simulink model "PL1_P2_PositionControl"  (R2022b)
settings: Solver=VariableStepAuto  StartTime=0.0  StopTime=10.0  RelTol=1e-3
values from neighbouring files (symbols this model uses):
  refx = rand    [RunPositionControl.m]
  refy = rand    [RunPositionControl.m]
undefined symbols (not defined in the file or in its folder): DiscIntNeverNeededParam
settings Model: Creator=lucas  LastModifiedBy=lucas
settings DataIOCC: ReturnWorkspaceOutputs=off

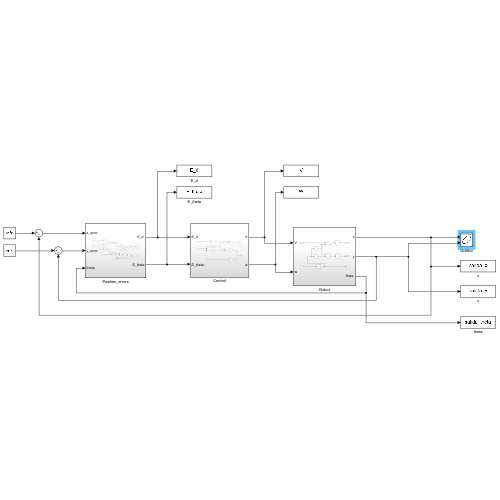
[thumbnail: Simulink's stored preview of the top-level diagram]
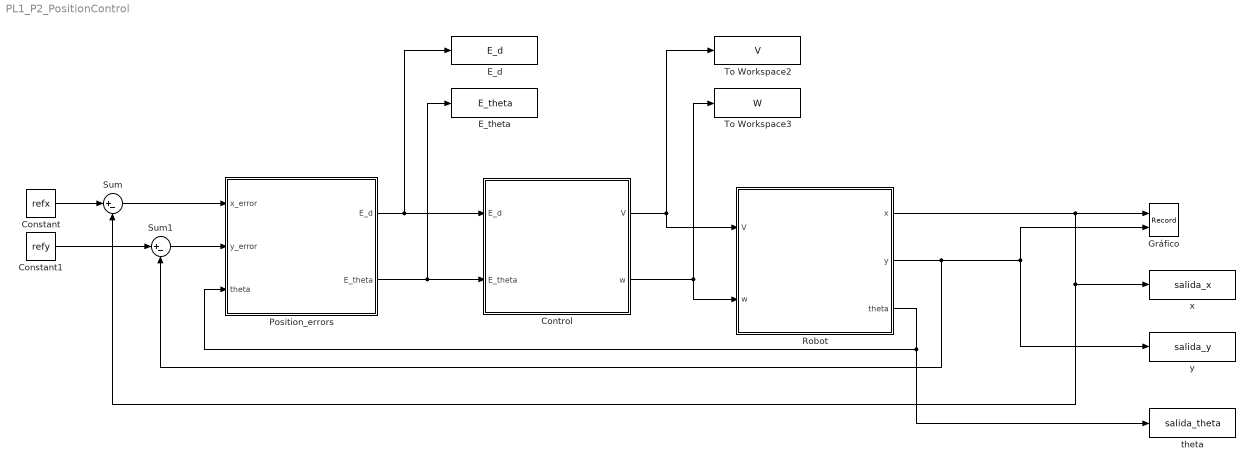
== system PL1_P2_PositionControl ==
  Constant : Constant  Value=refx
  Constant1 : Constant  Value=refy
  Control : Subsystem
  E_d : ToWorkspace  VariableName=E_d  SaveFormat=Structure With Time  SampleTime=-1
  E_theta : ToWorkspace  VariableName=E_theta  SaveFormat=Structure With Time  SampleTime=-1
  Gráfico : Record  FileSettingsInternal="{\"entries\":[{\"content\":{\"excelSettings\":{\"content\":{},\"type\":\"Streamout.ExcelSettings\"}},\"type\":\"Streamout.FileSettingStorage\",\"uuid\":\"\"}],\"packageUris\":[\"http:\\/\\/schema.mathworks.com\\/mf0\\/streamout_blocks\\/R2020a\"],\"version\":\"1.0\"}"  Layout=[1 1]  SignalsInternal="{\"entries\":[{\"content\":{\"signals\":[{\"content\":{\"blockPath\":[],\"channel\":[],\"dimensions\":[1],\"domain\":\"\",\"lineColor\":\"#0072bd\",\"plots\":[1],\"port\":1,\"sid\":[\"\"],\"signalID\":2497,\"signalName\":\"Robot:1\"},\"type\":\"RecordBlkView.Signal\",\"uuid\":\"\"},{\"content\":{\"blockPath\":[],\"channel\":[],\"dimensions\":[1],\"domain\":\"\",\"lineColor\":\"#d95319\",\"plots\":[1],\"port\":2,\"sid\":[\"\"],\"signalID\":2501,\"signalName\":\"Robot:2\"},\"type\":\"RecordBlkView.Signal\",\"uuid\":\"\"}]},\"type\":\"RecordBlkView.InputSignals\",\"uuid\":\"\"}],\"packageUris\":[\"http:\\/\\/schema.mathworks.com\\/mf0\\/streamout_blocks\\/R2020a\"],\"version\":\"1.0\"}"  VisualizationBindings="{\"xyplotplugin\":{\"info\":[{\"series\":[{\"bindingParametersList\":[{\"parameter\":\"X-Axis\",\"signalID\":2497,\"signalName\":\"Robot:1\"},{\"parameter\":\"Y-Axis\",\"signalID\":2501,\"signalName\":\"Robot:2\"}],\"seriesID\":28655},{\"bindingParametersList\":[{\"parameter\":\"X-Axis\",\"signalID\":2501,\"signalName\":\"Robot:2\"},{\"parameter\":\"Y-Axis\",\"signalID\":2497,\"signalName\":\"Robot:1\"}],\"seriesID\":47687}],\"subplotID\":1}]}}"  CompatibilityTag=XY  st=-1
  Position_errors : Subsystem
  Robot : Subsystem
  Sum : Sum  Inputs=|+-
  Sum1 : Sum  Inputs=|+-
  To Workspace2 : ToWorkspace  VariableName=V  SaveFormat=Structure With Time  SampleTime=-1
  To Workspace3 : ToWorkspace  VariableName=W  SaveFormat=Structure With Time  SampleTime=-1
  theta : ToWorkspace  VariableName=salida_theta  SaveFormat=Structure With Time  SampleTime=-1
  x : ToWorkspace  VariableName=salida_x  SaveFormat=Structure With Time  SampleTime=-1
  y : ToWorkspace  VariableName=salida_y  SaveFormat=Structure With Time  SampleTime=-1
  wires:
  Position_errors/2(E_theta) -> Control/2(E_theta), E_theta/1
  Control/2(w) -> To Workspace3/1, Robot/2(w)
  Constant1/1 -> Sum1/1
  Constant/1 -> Sum/1
  Sum/1 -> Position_errors/1("x_error ")
  Sum1/1 -> Position_errors/2("y_error ")
  Position_errors/1("E_d ") -> E_d/1, Control/1(E_d)
  Control/1(V) -> Robot/1(V), To Workspace2/1
  Robot/1(x) -> Sum/2, x/1, Gráfico/1
  Robot/2(y) -> Sum1/2, Gráfico/2, y/1
  Robot/3("theta ") -> Position_errors/3(theta), theta/1

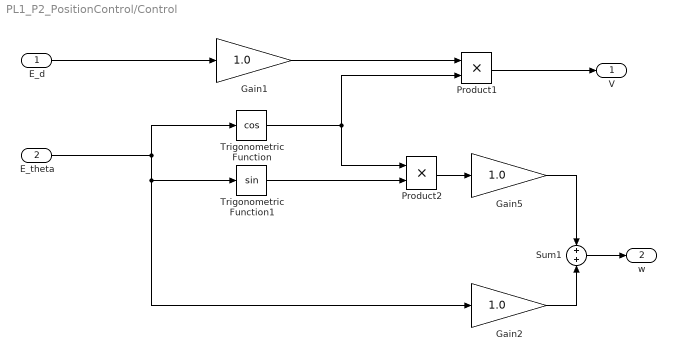
== system PL1_P2_PositionControl/Control ==
  E_d : Inport
  E_theta : Inport  Port=2
  Gain1 : Gain  Gain=1.0
  Gain2 : Gain  Gain=1.0
  Gain5 : Gain  Gain=1.0
  Product1 : Product
  Product2 : Product
  Sum1 : Sum
  Trigonometric Function : Trigonometry  Operator=cos
  Trigonometric Function1 : Trigonometry
  V : Outport  VectorParamsAs1DForOutWhenUnconnected=off
  w : Outport  Port=2  VectorParamsAs1DForOutWhenUnconnected=off
  wires:
  Sum1/1 -> w/1
  Gain2/1 -> Sum1/2
  Gain5/1 -> Sum1/1
  Gain1/1 -> Product1/1
  Product2/1 -> Gain5/1
  Trigonometric Function1/1 -> Product2/2
  Product1/1 -> V/1
  Trigonometric Function/1 -> Product2/1, Product1/2
  E_d/1 -> Gain1/1
  E_theta/1 -> Trigonometric Function/1, Trigonometric Function1/1, Gain2/1

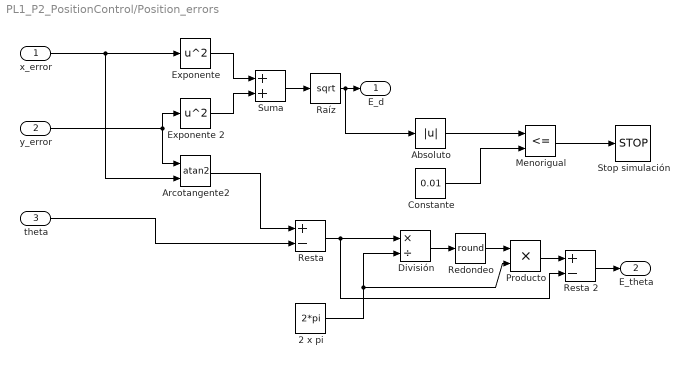
== system PL1_P2_PositionControl/Position_errors ==
  "x_error " : Inport
  "y_error " : Inport  Port=2
  theta : Inport  Port=3
  2 x pi : Constant  Value=2*pi
  Absoluto : Abs  SaturateOnIntegerOverflow=off
  Arcotangente2 : Trigonometry  Operator=atan2
  Constante : Constant  Value=0.01
  División : Product  Inputs=*/
  Exponente : Math  Operator=square
  Exponente 2 : Math  Operator=square
  Menorigual : RelationalOperator  Operator=<=  OutDataTypeStr=boolean  RndMeth=Simplest  InputSameDT=off
  Producto : Product
  Raíz : Sqrt
  Redondeo : Rounding  Operator=round
  Resta : Sum  Inputs=+-  OutMin=[-pi]  OutMax=[pi]
  Resta 2 : Sum  Inputs=+-  OutMin=[-pi]  OutMax=[pi]
  Stop simulación : Stop
  Suma : Sum
  "E_d " : Outport
  E_theta : Outport  Port=2
  wires:
  theta/1 -> Resta/2
  "y_error "/1 -> Exponente 2/1, Arcotangente2/1
  Arcotangente2/1 -> Resta/1
  Menorigual/1 -> Stop simulación/1
  Suma/1 -> Raíz/1
  Exponente 2/1 -> Suma/2
  Raíz/1 -> "E_d "/1, Absoluto/1
  Constante/1 -> Menorigual/2
  División/1 -> Redondeo/1
  Redondeo/1 -> Producto/1
  Absoluto/1 -> Menorigual/1
  "x_error "/1 -> Exponente/1, Arcotangente2/2
  Exponente/1 -> Suma/1
  2 x pi/1 -> División/2, Producto/2
  Producto/1 -> Resta 2/1
  Resta/1 -> División/1, Resta 2/2
  Resta 2/1 -> E_theta/1

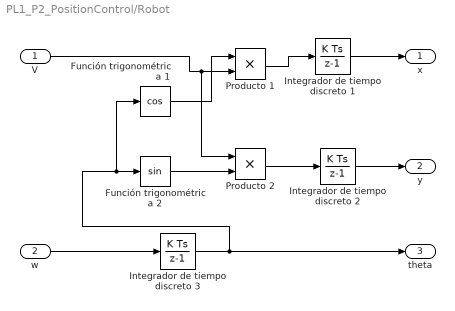
== system PL1_P2_PositionControl/Robot ==
  V : Inport
  w : Inport  Port=2
  Función trigonométrica 1 : Trigonometry  Operator=cos
  Función trigonométrica 2 : Trigonometry
  Integrador de tiempo discreto 1 : DiscreteIntegrator  InitialCondition=-4  SampleTime=0.01  ICPrevOutput=DiscIntNeverNeededParam  ICPrevScaledInput=DiscIntNeverNeededParam
  Integrador de tiempo discreto 2 : DiscreteIntegrator  InitialCondition=-4  SampleTime=0.01  ICPrevOutput=DiscIntNeverNeededParam  ICPrevScaledInput=DiscIntNeverNeededParam
  Integrador de tiempo discreto 3 : DiscreteIntegrator  SampleTime=0.01  ICPrevOutput=DiscIntNeverNeededParam  ICPrevScaledInput=DiscIntNeverNeededParam
  Producto 1 : Product
  Producto 2 : Product
  x : Outport  VectorParamsAs1DForOutWhenUnconnected=off
  y : Outport  Port=2  VectorParamsAs1DForOutWhenUnconnected=off
  "theta " : Outport  Port=3  VectorParamsAs1DForOutWhenUnconnected=off
  wires:
  V/1 -> Producto 2/1, Producto 1/2
  Integrador de tiempo discreto 2/1 -> y/1
  Producto 1/1 -> Integrador de tiempo discreto 1/1
  w/1 -> Integrador de tiempo discreto 3/1
  Función trigonométrica 2/1 -> Producto 2/2
  Producto 2/1 -> Integrador de tiempo discreto 2/1
  Integrador de tiempo discreto 3/1 -> "theta "/1, Función trigonométrica 1/1, Función trigonométrica 2/1
  Integrador de tiempo discreto 1/1 -> x/1
  Función trigonométrica 1/1 -> Producto 1/1
